simulink model "test_2"  (R2024b)
settings: Solver=FixedStepAuto  StartTime=0.0  StopTime=100000  RelTol=1e-3  EnableMultiTasking=on
undefined symbols (not defined in the file): BOOL, DINT, OTL, slplc
libraries: arduinolib x4
(part 1 of 8)
settings Model: ExtModeTrigDuration=2  Creator=Elliot  LastModifiedBy=Elliot
settings SolverCC: AutoInsertRateTranBlk=on
settings OptimizationCC: EnhancedBackFolding=on  PassReuseOutputArgsAs=Individual arguments  ZeroExternalMemoryAtStartup=off  ZeroInternalMemoryAtStartup=off  MaxStackSize=64  OptimizeBlockOrder=speed  DifferentSizesBufferReuse=on  OptimizationCustomize=off  EfficientTunableParamExpr=on
settings DebuggingCC: ParameterTunabilityLossMsg=error
settings HardwareCC: ProdBitPerInt=16  ProdBitPerPointer=16  ProdBitPerSizeT=16  ProdBitPerPtrDiffT=16  ProdLargestAtomicFloat=None  ProdWordSize=8  ProdHWDeviceType=Atmel->AVR
settings SFSimCC: MATLABDynamicMemAlloc=off
settings RTWCC: Description=Embedded Coder  SystemTargetFile=ert.tlc  HardwareBoard=Arduino Uno  TemplateMakefile=ert_default_tmf  Toolchain=Arduino AVR  BuildConfiguration=Faster Runs
settings CodeAppCC: ForceParamTrailComments=on  IgnoreCustomStorageClasses=off  OperatorAnnotations=on  SimulinkDataObjDesc=on  SFDataObjDesc=on  InsertBlockDesc=on
settings ERTTargetCC: SupportContinuousTime=on  SupportVariableSizeSignals=on  ExtModeTransport=3  ExtModeStaticAlloc=on  ExtModeAutomaticAllocSize=off  ExtModeStaticAllocSize=250  ExtModeMexFile=ext_xcp  ExtModeIntrfLevel=Level2 - Open  InlinedParameterPlacement=Hierarchical

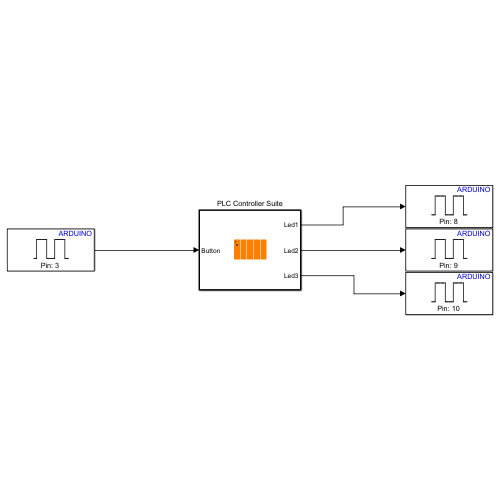
[thumbnail: Simulink's stored preview of the top-level diagram]
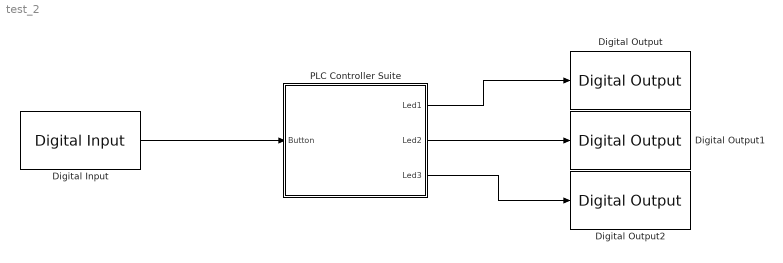
== system test_2 ==
  Digital Input : arduinolib/Digital Input  pinNumber=3  mode=Default  Direction=input  SampleTime=0.1  blockPlatform=arduino
  Digital Output : arduinolib/Digital Output  pinNumber=8  Direction=output  blockPlatform=arduino
  Digital Output1 : arduinolib/Digital Output  pinNumber=9  Direction=output  blockPlatform=arduino
  Digital Output2 : arduinolib/Digital Output  pinNumber=10  Direction=output  blockPlatform=arduino
  PLC Controller Suite : Subsystem  TreatAsAtomicUnit=on  mask{PLCBlockType=PLCController, PLCPOUType=PLC Controller}
      mask init:
      | slplc.callbacks.initController(gcb);
      settings: OpenFcn=slplc.callbacks.openPOUBlock(gcb);
      mask Help: web([docroot '/plccoder/ref/plccontrollersuite' '.html']);
      mask DialogControl PLCBlockTitle Prompt: PLC Controller Block
  wires:
  PLC Controller Suite/1(Led1) -> Digital Output/1
  PLC Controller Suite/2(Led2) -> Digital Output1/1
  PLC Controller Suite/3(Led3) -> Digital Output2/1
  Digital Input/1 -> PLC Controller Suite/1(Button)

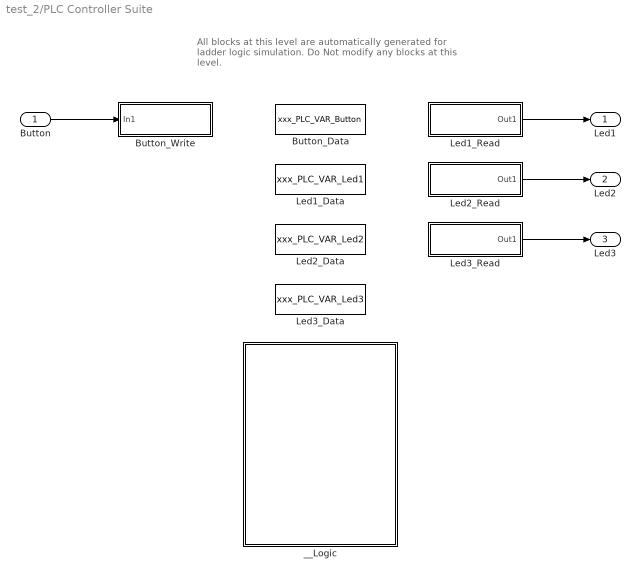
== system test_2/PLC Controller Suite ==
  note: All blocks at this level are automatically generated for ladder logic simulation.
      | Do Not modify any blocks at this level.
  Button : Inport  OutDataTypeStr=boolean
  Button_Data : DataStoreMemory  Tag=POUVariable  Priority=10  DataStoreName=xxx_PLC_VAR_Button  ShowAdditionalParam=off  OutDataTypeStr=boolean  Dimensions=1
  Button_Write : Subsystem  Priority=11  DisableCoverage=on  TreatAsAtomicUnit=on  mask{PLCOperandTag=Button, PLCOperandExpression=xxx_PLC_VAR_Button, PLCBlockType=VarWrite, PLCPOUType=VarWrite}
      mask prompts: PLCOperandTag "Operand Tag:"
      mask init:
      | slplc.callbacks.initInstruction(gcb);
      mask Help: web([docroot '/plccoder/ref/varwrite' '.html']);
      mask DialogControl PLCBlockTitle Prompt: Variable Write
      mask Display: disp(get_param(gcb, 'PLCOperandTag'));
  Led1_Data : DataStoreMemory  Tag=POUVariable  Priority=10  DataStoreName=xxx_PLC_VAR_Led1  ShowAdditionalParam=off  OutDataTypeStr=boolean  Dimensions=1
  Led1_Read : Subsystem  Priority=13  DisableCoverage=on  TreatAsAtomicUnit=on  mask{PLCOperandTag=Led1, PLCOperandExpression=xxx_PLC_VAR_Led1, PLCBlockType=VarRead, PLCPOUType=VarRead}
      mask prompts: PLCOperandTag "Operand Tag"
      mask init:
      | block = gcb;
      | maskObj = Simulink.Mask.get(block);
      | maskObj.Display = sprintf('disp(''%s'');', PLCOperandTag);
      | slplc.callbacks.initInstruction(gcb);
      mask Help: web([docroot '/plccoder/ref/varread' '.html']);
      mask DialogControl PLCBlockTitle Prompt: Variable Read
      mask Display: disp('Led1');
  Led2_Data : DataStoreMemory  Tag=POUVariable  Priority=10  DataStoreName=xxx_PLC_VAR_Led2  ShowAdditionalParam=off  OutDataTypeStr=boolean  Dimensions=1
  Led2_Read : Subsystem  Priority=13  DisableCoverage=on  TreatAsAtomicUnit=on  mask{PLCOperandTag=Led2, PLCOperandExpression=xxx_PLC_VAR_Led2, PLCBlockType=VarRead, PLCPOUType=VarRead}
      mask prompts: PLCOperandTag "Operand Tag"
      mask init:
      | block = gcb;
      | maskObj = Simulink.Mask.get(block);
      | maskObj.Display = sprintf('disp(''%s'');', PLCOperandTag);
      | slplc.callbacks.initInstruction(gcb);
      mask Help: web([docroot '/plccoder/ref/varread' '.html']);
      mask DialogControl PLCBlockTitle Prompt: Variable Read
      mask Display: disp('Led2');
  Led3_Data : DataStoreMemory  Tag=POUVariable  Priority=10  DataStoreName=xxx_PLC_VAR_Led3  ShowAdditionalParam=off  OutDataTypeStr=boolean  Dimensions=1
  Led3_Read : Subsystem  Priority=13  DisableCoverage=on  TreatAsAtomicUnit=on  mask{PLCOperandTag=Led3, PLCOperandExpression=xxx_PLC_VAR_Led3, PLCBlockType=VarRead, PLCPOUType=VarRead}
      mask prompts: PLCOperandTag "Operand Tag"
      mask init:
      | block = gcb;
      | maskObj = Simulink.Mask.get(block);
      | maskObj.Display = sprintf('disp(''%s'');', PLCOperandTag);
      | slplc.callbacks.initInstruction(gcb);
      mask Help: web([docroot '/plccoder/ref/varread' '.html']);
      mask DialogControl PLCBlockTitle Prompt: Variable Read
      mask Display: disp('Led3');
  __Logic : Subsystem  Priority=12  TreatAsAtomicUnit=on
  Led1 : Outport
  Led2 : Outport  Port=2
  Led3 : Outport  Port=3
  wires:
  Button/1 -> Button_Write/1(In1)
  Led1_Read/1(Out1) -> Led1/1
  Led2_Read/1(Out1) -> Led2/1
  Led3_Read/1(Out1) -> Led3/1

== system test_2/PLC Controller Suite/Button_Write ==
  In1 : Inport
  __CoreVarWrite : Subsystem  Tag=CoreVarWriteBlock  DisableCoverage=on  TreatAsAtomicUnit=on  mask{PLCBlockType=CoreVarWrite}
      mask init:
      | slplc.callbacks.initCoreVariable(gcb, 'write');
      mask DialogControl PLCBlockTitle Prompt: Core Variable Write
  wires:
  In1/1 -> __CoreVarWrite/1(u)

== system test_2/PLC Controller Suite/Led1_Read ==
  __CoreVarRead : Subsystem  Tag=CoreVarReadBlock  DisableCoverage=on  TreatAsAtomicUnit=on  mask{PLCBlockType=CoreVarRead}
      mask init:
      | slplc.callbacks.initCoreVariable(gcb, 'read');
      mask DialogControl PLCBlockTitle Prompt: Core Variable Read
  Out1 : Outport  VectorParamsAs1DForOutWhenUnconnected=off
  wires:
  __CoreVarRead/1(y) -> Out1/1

== system test_2/PLC Controller Suite/Led2_Read ==
  __CoreVarRead : Subsystem  Tag=CoreVarReadBlock  DisableCoverage=on  TreatAsAtomicUnit=on  mask{PLCBlockType=CoreVarRead}
      mask init:
      | slplc.callbacks.initCoreVariable(gcb, 'read');
      mask DialogControl PLCBlockTitle Prompt: Core Variable Read
  Out1 : Outport  VectorParamsAs1DForOutWhenUnconnected=off
  wires:
  __CoreVarRead/1(y) -> Out1/1

== system test_2/PLC Controller Suite/Led3_Read ==
  __CoreVarRead : Subsystem  Tag=CoreVarReadBlock  DisableCoverage=on  TreatAsAtomicUnit=on  mask{PLCBlockType=CoreVarRead}
      mask init:
      | slplc.callbacks.initCoreVariable(gcb, 'read');
      mask DialogControl PLCBlockTitle Prompt: Core Variable Read
  Out1 : Outport  VectorParamsAs1DForOutWhenUnconnected=off
  wires:
  __CoreVarRead/1(y) -> Out1/1

== system test_2/PLC Controller Suite/__Logic ==
  Controller Tags : Subsystem  Tag=ControllerVariableSS  DisableCoverage=on  TreatAsAtomicUnit=on  mask{PLCVarButtonName=Button, PLCVarButtonAddress=<empty>, PLCVarButtonMapping=Input Symbol, PLCVarButtonPortIndex=1, PLCVarButtonDataType=boolean, PLCVarButtonSize=1, PLCVarButtonInitialValue=0, PLCVarButtonToDelete=off, PLCVarLed1Name=Led1, PLCVarLed1Address=<empty>, PLCVarLed1Mapping=Output Symbol, PLCVarLed1PortIndex=1, PLCVarLed1DataType=boolean, PLCVarLed1Size=1, PLCVarLed1InitialValue=0, PLCVarLed1ToDelete=off, PLCVarLed2Name=Led2, PLCVarLed2Address=<empty>, PLCVarLed2Mapping=Output Symbol, PLCVarLed2PortIndex=2, PLCVarLed2DataType=boolean, PLCVarLed2Size=1, PLCVarLed2InitialValue=0, PLCVarLed2ToDelete=off, PLCVarLed3Name=Led3, PLCVarLed3Address=<empty>, PLCVarLed3Mapping=Output Symbol, PLCVarLed3PortIndex=3, PLCVarLed3DataType=boolean, PLCVarLed3Size=1, PLCVarLed3InitialValue=0, PLCVarLed3ToDelete=off}
      mask init:
      | slplc.callbacks.initControllerVarSS(gcb);
      settings: OpenFcn=slplc.callbacks.openControllerVariableSS(gcb);
      mask Help: web([docroot '/plccoder/ref/controllertags' '.html']);
      mask TypeOptions PLCVarButtonMapping: Global Variable | Input Symbol | Output Symbol
      mask TypeOptions PLCVarButtonPortIndex: 1 | 2 | 3 | 4
      mask TypeOptions PLCVarLed1Mapping: Global Variable | Input Symbol | Output Symbol
      mask TypeOptions PLCVarLed1PortIndex: 1 | 2 | 3 | 4
      mask TypeOptions PLCVarLed2Mapping: Global Variable | Input Symbol | Output Symbol
      mask TypeOptions PLCVarLed2PortIndex: 1 | 2 | 3 | 4
      mask TypeOptions PLCVarLed3Mapping: Global Variable | Input Symbol | Output Symbol
      mask TypeOptions PLCVarLed3PortIndex: 1 | 2 | 3 | 4
      mask DialogControl PLCBlockTitle Prompt: Global Variable and Symbol Spreadsheet
      mask DialogControl PLCVarListHeaderName Prompt: Name
      mask DialogControl PLCVarListHeaderAddress Prompt: Address (At)
      mask DialogControl PLCVarListHeaderMapping Prompt: Mapping Type
      mask DialogControl PLCVarListHeaderPortIndex Prompt: Port
      mask DialogControl PLCVarListHeaderDataType Prompt: Data Type
      mask DialogControl PLCVarListHeaderSize Prompt: Size
      mask DialogControl PLCVarListHeaderInitialValue Prompt: Initial Value
      mask DialogControl PLCVarListHeaderToDelete Prompt: Delete
  Task : Subsystem  TreatAsAtomicUnit=on  mask{PLCBlockType=Task, PLCPOUType=Task, PLCTaskWatchDog=0}
      settings: OpenFcn=slplc.callbacks.openTaskBlock(gcb);
      mask Help: web([docroot '/plccoder/ref/task' '.html']);
      mask DialogControl PLCBlockTitle Prompt: Task
  Up to Parent POU : Subsystem  DisableCoverage=on  TreatAsAtomicUnit=on  mask{PLCBlockType=OpenParentPOU}
      settings: OpenFcn=slplc.callbacks.openParentPOUBlock(gcb);
      mask Help: web([docroot '/plccoder/ref/uptoparentpou' '.html']);
      mask DialogControl PLCBlockTitle Prompt: Add Single Rung

== system test_2/PLC Controller Suite/Button_Write/__CoreVarWrite ==
  u : Inport
  DataWrite : DataStoreWrite  DataStoreName=xxx_PLC_VAR_Button  IndexOptions=Index vector (dialog)  Indices=1  OutputSizes=1
  wires:
  u/1 -> DataWrite/1

== system test_2/PLC Controller Suite/Led1_Read/__CoreVarRead ==
  DataRead : DataStoreRead  DataStoreName=xxx_PLC_VAR_Led1  IndexOptions=Index vector (dialog)  Indices=1  OutputSizes=1
  y : Outport  VectorParamsAs1DForOutWhenUnconnected=off
  wires:
  DataRead/1 -> y/1

== system test_2/PLC Controller Suite/Led2_Read/__CoreVarRead ==
  DataRead : DataStoreRead  DataStoreName=xxx_PLC_VAR_Led2  IndexOptions=Index vector (dialog)  Indices=1  OutputSizes=1
  y : Outport  VectorParamsAs1DForOutWhenUnconnected=off
  wires:
  DataRead/1 -> y/1

== system test_2/PLC Controller Suite/Led3_Read/__CoreVarRead ==
  DataRead : DataStoreRead  DataStoreName=xxx_PLC_VAR_Led3  IndexOptions=Index vector (dialog)  Indices=1  OutputSizes=1
  y : Outport  VectorParamsAs1DForOutWhenUnconnected=off
  wires:
  DataRead/1 -> y/1

== system test_2/PLC Controller Suite/__Logic/Controller Tags ==

== system test_2/PLC Controller Suite/__Logic/Task ==
  Program : Subsystem  TreatAsAtomicUnit=on  mask{PLCPOUType=Program, PLCPOULanguage=LD, PLCBlockType=LDProgram}
      mask prompts: PLCPOUType "POU Type:"
      mask init:
      | slplc.callbacks.initProgram(gcb);
      settings: OpenFcn=slplc.callbacks.openPOUBlock(gcb);
      mask Help: web([docroot '/plccoder/ref/ldprogram' '.html']);
      mask DialogControl PLCBlockTitle Prompt: Program
      mask DialogControl PLCEditPOU Prompt: Edit POU
      mask DialogControl PLCEditInterface Prompt: Edit Variables
  Up to Parent POU : Subsystem  DisableCoverage=on  TreatAsAtomicUnit=on  mask{PLCBlockType=OpenParentPOU}
      settings: OpenFcn=slplc.callbacks.openParentPOUBlock(gcb);
      mask Help: web([docroot '/plccoder/ref/uptoparentpou' '.html']);
      mask DialogControl PLCBlockTitle Prompt: Add Single Rung

== system test_2/PLC Controller Suite/__Logic/Up to Parent POU ==

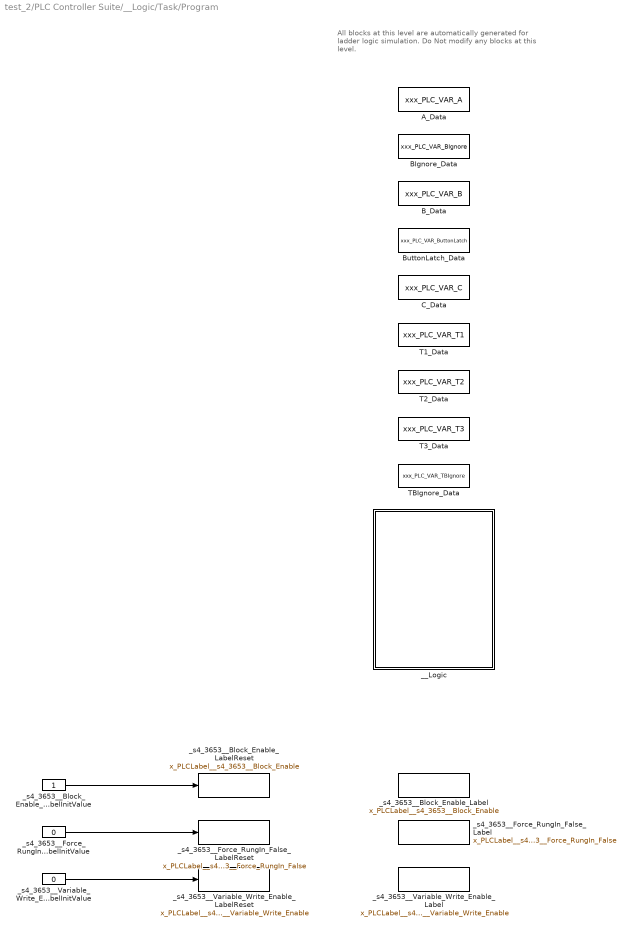
== system test_2/PLC Controller Suite/__Logic/Task/Program ==
  note: All blocks at this level are automatically generated for ladder logic simulation.
      | Do Not modify any blocks at this level.
  A_Data : DataStoreMemory  Tag=POUVariable  Priority=10  DataStoreName=xxx_PLC_VAR_A  InitialValue=true  ShowAdditionalParam=off  OutDataTypeStr=BOOL  Dimensions=1
  BIgnore_Data : DataStoreMemory  Tag=POUVariable  Priority=10  DataStoreName=xxx_PLC_VAR_BIgnore  InitialValue=false  ShowAdditionalParam=off  OutDataTypeStr=BOOL  Dimensions=1
  B_Data : DataStoreMemory  Tag=POUVariable  Priority=10  DataStoreName=xxx_PLC_VAR_B  InitialValue=false  ShowAdditionalParam=off  OutDataTypeStr=BOOL  Dimensions=1
  ButtonLatch_Data : DataStoreMemory  Tag=POUVariable  Priority=10  DataStoreName=xxx_PLC_VAR_ButtonLatch  InitialValue=false  ShowAdditionalParam=off  OutDataTypeStr=BOOL  Dimensions=1
  C_Data : DataStoreMemory  Tag=POUVariable  Priority=10  DataStoreName=xxx_PLC_VAR_C  InitialValue=false  ShowAdditionalParam=off  OutDataTypeStr=BOOL  Dimensions=1
  T1_Data : DataStoreMemory  Tag=POUVariable  Priority=10  DataStoreName=xxx_PLC_VAR_T1  InitialValue=T1_InitialValue  ShowAdditionalParam=off  OutDataTypeStr=Bus: TIMER  Dimensions=1
  T2_Data : DataStoreMemory  Tag=POUVariable  Priority=10  DataStoreName=xxx_PLC_VAR_T2  InitialValue=T1_InitialValue  ShowAdditionalParam=off  OutDataTypeStr=Bus: TIMER  Dimensions=1
  T3_Data : DataStoreMemory  Tag=POUVariable  Priority=10  DataStoreName=xxx_PLC_VAR_T3  InitialValue=T1_InitialValue  ShowAdditionalParam=off  OutDataTypeStr=Bus: TIMER  Dimensions=1
  TBIgnore_Data : DataStoreMemory  Tag=POUVariable  Priority=10  DataStoreName=xxx_PLC_VAR_TBIgnore  InitialValue=T2_InitialValue  ShowAdditionalParam=off  OutDataTypeStr=Bus: TIMER  Dimensions=1
  __Logic : Subsystem  Priority=12  TreatAsAtomicUnit=on
  _s4_3653__Block_Enable_Label : DataStoreMemory  Priority=10  DataStoreName=x_PLCLabel__s4_3653__Block_Enable  InitialValue=1  ShowAdditionalParam=off  OutDataTypeStr=BOOL  Dimensions=1
  _s4_3653__Block_Enable_LabelInitValue : Constant  OutDataTypeStr=BOOL
  _s4_3653__Block_Enable_LabelReset : DataStoreWrite  Priority=11  DataStoreName=x_PLCLabel__s4_3653__Block_Enable  IndexOptions=Index vector (dialog)  Indices=1  OutputSizes=1
  _s4_3653__Force_RungIn_False_Label : DataStoreMemory  Priority=10  DataStoreName=x_PLCLabel__s4_3653__Force_RungIn_False  ShowAdditionalParam=off  OutDataTypeStr=BOOL  Dimensions=1
  _s4_3653__Force_RungIn_False_LabelInitValue : Constant  Value=0  OutDataTypeStr=BOOL
  _s4_3653__Force_RungIn_False_LabelReset : DataStoreWrite  Priority=11  DataStoreName=x_PLCLabel__s4_3653__Force_RungIn_False  IndexOptions=Index vector (dialog)  Indices=1  OutputSizes=1
  _s4_3653__Variable_Write_Enable_Label : DataStoreMemory  Priority=10  DataStoreName=x_PLCLabel__s4_3653__Variable_Write_Enable  ShowAdditionalParam=off  OutDataTypeStr=BOOL  Dimensions=1
  _s4_3653__Variable_Write_Enable_LabelInitValue : Constant  Value=0  OutDataTypeStr=BOOL
  _s4_3653__Variable_Write_Enable_LabelReset : DataStoreWrite  Priority=11  DataStoreName=x_PLCLabel__s4_3653__Variable_Write_Enable  IndexOptions=Index vector (dialog)  Indices=1  OutputSizes=1
  wires:
  _s4_3653__Block_Enable_LabelInitValue/1 -> _s4_3653__Block_Enable_LabelReset/1
  _s4_3653__Variable_Write_Enable_LabelInitValue/1 -> _s4_3653__Variable_Write_Enable_LabelReset/1
  _s4_3653__Force_RungIn_False_LabelInitValue/1 -> _s4_3653__Force_RungIn_False_LabelReset/1

== system test_2/PLC Controller Suite/__Logic/Task/Up to Parent POU ==

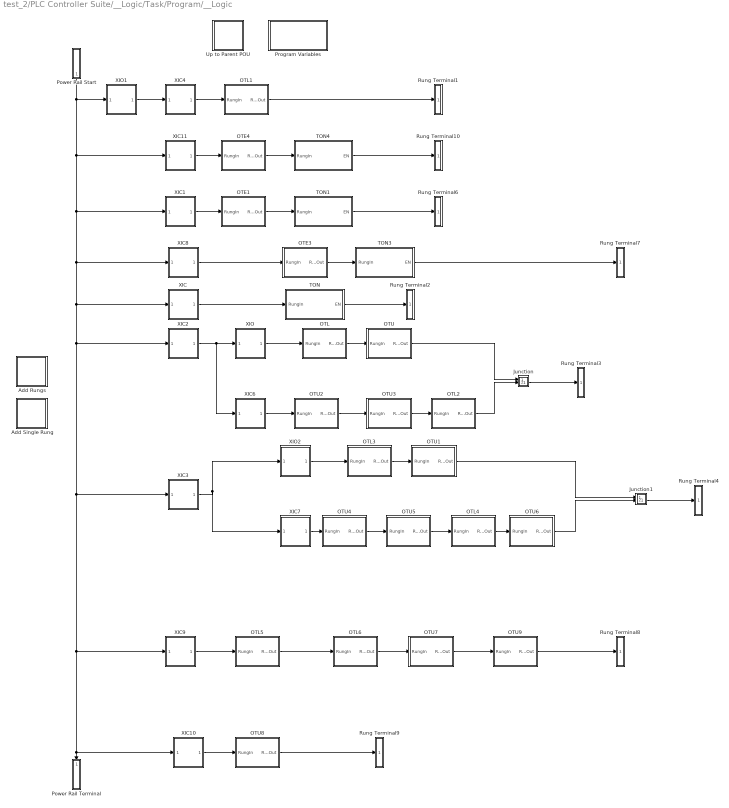
== system test_2/PLC Controller Suite/__Logic/Task/Program/__Logic ==
  Add Rungs : Subsystem  DisableCoverage=on  TreatAsAtomicUnit=on  mask{PLCRungNumberToAdd=1, PLCBlockType=AddRungs}
      mask prompts: PLCRungNumberToAdd "Rung Number:"
      mask Help: web([docroot '/plccoder/ref/addrungs' '.html']);
      mask DialogControl PLCAddRungs Prompt: Add Rungs
      mask DialogControl PLCRungAddButton Prompt: Add
      mask DialogControl PLCRungAddButton Callback: slplc.callbacks.addLadderRungs(gcb);
      mask Display: disp(sprintf(['Add' newline 'Rungs']));
  Add Single Rung : Subsystem  DisableCoverage=on  TreatAsAtomicUnit=on  mask{PLCRungNumberToAdd=1, PLCBlockType=AddSingleRung}
      settings: OpenFcn=slplc.callbacks.addLadderRungs(gcb);
      mask Help: web([docroot '/plccoder/ref/addsinglerung' '.html']);
      mask DialogControl PLCAddRung Prompt: Add Single Rung
      mask Display: disp(sprintf(['Add' newline '1 Rung']));
  Junction : Subsystem  Priority=29  DisableCoverage=on  TreatAsAtomicUnit=on  mask{PLCBlockType=Junction, PLCPOUType=BranchJunction}
      mask Help: web([docroot '/plccoder/ref/junction' '.html']);
      mask DialogControl PLCBlockTitle Prompt: Rung Merge Point
      mask DialogControl PLCBlockDesc Prompt: This is the ladder diagram rung merge point.
  Junction1 : Subsystem  Priority=40  DisableCoverage=on  TreatAsAtomicUnit=on  mask{PLCBlockType=Junction, PLCPOUType=BranchJunction}
      mask Help: web([docroot '/plccoder/ref/junction' '.html']);
      mask DialogControl PLCBlockTitle Prompt: Rung Merge Point
      mask DialogControl PLCBlockDesc Prompt: This is the ladder diagram rung merge point.
  OTE1 : Subsystem  Priority=11  TreatAsAtomicUnit=on  mask{PLCOperandTag=Led2, PLCBlockType=OTE, PLCPOUType=Coil, PLCOperandExpression=xxx_PLC_VAR_Led2}
      mask prompts: PLCOperandTag "Operand Tag:"
      mask init:
      | slplc.callbacks.initInstruction(gcb);
      settings: AttributesFormatString=%<PLCOperandTag>
      mask Help: web([docroot '/plccoder/ref/ote' '.html']);
      mask DialogControl PLCBlockTitle Prompt: Output Energize (OTE)
  OTE3 : Subsystem  Priority=15  TreatAsAtomicUnit=on  mask{PLCOperandTag=Led3, PLCBlockType=OTE, PLCPOUType=Coil, PLCOperandExpression=xxx_PLC_VAR_Led3}
      mask prompts: PLCOperandTag "Operand Tag:"
      mask init:
      | slplc.callbacks.initInstruction(gcb);
      settings: AttributesFormatString=%<PLCOperandTag>
      mask Help: web([docroot '/plccoder/ref/ote' '.html']);
      mask DialogControl PLCBlockTitle Prompt: Output Energize (OTE)
  OTE4 : Subsystem  Priority=7  TreatAsAtomicUnit=on  mask{PLCOperandTag=Led1, PLCBlockType=OTE, PLCPOUType=Coil, PLCOperandExpression=xxx_PLC_VAR_Led1}
      mask prompts: PLCOperandTag "Operand Tag:"
      mask init:
      | slplc.callbacks.initInstruction(gcb);
      settings: AttributesFormatString=%<PLCOperandTag>
      mask Help: web([docroot '/plccoder/ref/ote' '.html']);
      mask DialogControl PLCBlockTitle Prompt: Output Energize (OTE)
  OTL : Subsystem  Priority=23  TreatAsAtomicUnit=on  mask{PLCOperandTag=B, PLCBlockType=OTL, PLCPOUType=Coil, PLCOperandExpression=xxx_PLC_VAR_B}
      mask prompts: PLCOperandTag "Operand Tag:"
      mask init:
      | slplc.callbacks.initInstruction(gcb);
      settings: AttributesFormatString=%<PLCOperandTag>
      mask Help: web([docroot '/plccoder/ref/otl' '.html']);
      mask DialogControl PLCBlockTitle Prompt: Output Latch (OTL)
      mask Display: disp('L');
  OTL1 : Subsystem  Priority=4  TreatAsAtomicUnit=on  mask{PLCOperandTag=ButtonLatch, PLCBlockType=OTL, PLCPOUType=Coil, PLCOperandExpression=xxx_PLC_VAR_ButtonLatch}
      mask prompts: PLCOperandTag "Operand Tag:"
      mask init:
      | slplc.callbacks.initInstruction(gcb);
      settings: AttributesFormatString=%<PLCOperandTag>
      mask Help: web([docroot '/plccoder/ref/otl' '.html']);
      mask DialogControl PLCBlockTitle Prompt: Output Latch (OTL)
      mask Display: disp('L');
  OTL2 : Subsystem  Priority=28  TreatAsAtomicUnit=on  mask{PLCOperandTag=C, PLCBlockType=OTL, PLCPOUType=Coil, PLCOperandExpression=xxx_PLC_VAR_C}
      mask prompts: PLCOperandTag "Operand Tag:"
      mask init:
      | slplc.callbacks.initInstruction(gcb);
      settings: AttributesFormatString=%<PLCOperandTag>
      mask Help: web([docroot '/plccoder/ref/otl' '.html']);
      mask DialogControl PLCBlockTitle Prompt: Output Latch (OTL)
      mask Display: disp('L');
  OTL3 : Subsystem  Priority=33  TreatAsAtomicUnit=on  mask{PLCOperandTag=A, PLCBlockType=OTL, PLCPOUType=Coil, PLCOperandExpression=xxx_PLC_VAR_A}
      mask prompts: PLCOperandTag "Operand Tag:"
      mask init:
      | slplc.callbacks.initInstruction(gcb);
      settings: AttributesFormatString=%<PLCOperandTag>
      mask Help: web([docroot '/plccoder/ref/otl' '.html']);
      mask DialogControl PLCBlockTitle Prompt: Output Latch (OTL)
      mask Display: disp('L');
  OTL4 : Subsystem  Priority=38  TreatAsAtomicUnit=on  mask{PLCOperandTag=C, PLCBlockType=OTL, PLCPOUType=Coil, PLCOperandExpression=xxx_PLC_VAR_C}
      mask prompts: PLCOperandTag "Operand Tag:"
      mask init:
      | slplc.callbacks.initInstruction(gcb);
      settings: AttributesFormatString=%<PLCOperandTag>
      mask Help: web([docroot '/plccoder/ref/otl' '.html']);
      mask DialogControl PLCBlockTitle Prompt: Output Latch (OTL)
      mask Display: disp('L');
  OTL5 : Subsystem  Priority=43  TreatAsAtomicUnit=on  mask{PLCOperandTag=A, PLCBlockType=OTL, PLCPOUType=Coil, PLCOperandExpression=xxx_PLC_VAR_A}
      mask prompts: PLCOperandTag "Operand Tag:"
      mask init:
      | slplc.callbacks.initInstruction(gcb);
      settings: AttributesFormatString=%<PLCOperandTag>
      mask Help: web([docroot '/plccoder/ref/otl' '.html']);
      mask DialogControl PLCBlockTitle Prompt: Output Latch (OTL)
      mask Display: disp('L');
  OTL6 : Subsystem  Priority=44  TreatAsAtomicUnit=on  mask{PLCOperandTag=BIgnore, PLCBlockType=OTL, PLCPOUType=Coil, PLCOperandExpression=xxx_PLC_VAR_BIgnore}
      mask prompts: PLCOperandTag "Operand Tag:"
      mask init:
      | slplc.callbacks.initInstruction(gcb);
      settings: AttributesFormatString=%<PLCOperandTag>
      mask Help: web([docroot '/plccoder/ref/otl' '.html']);
      mask DialogControl PLCBlockTitle Prompt: Output Latch (OTL)
      mask Display: disp('L');
  OTU : Subsystem  Priority=24  TreatAsAtomicUnit=on  mask{PLCOperandTag=A, PLCBlockType=OTU, PLCPOUType=Coil, PLCOperandExpression=xxx_PLC_VAR_A}
      mask prompts: PLCOperandTag "Operand Tag:"
      mask init:
      | slplc.callbacks.initInstruction(gcb);
      settings: AttributesFormatString=%<PLCOperandTag>
      mask Help: web([docroot '/plccoder/ref/otu' '.html']);
      mask DialogControl PLCBlockTitle Prompt: Output Unlatch (OTU)
      mask Display: disp('U');
  OTU1 : Subsystem  Priority=34  TreatAsAtomicUnit=on  mask{PLCOperandTag=B, PLCBlockType=OTU, PLCPOUType=Coil, PLCOperandExpression=xxx_PLC_VAR_B}
      mask prompts: PLCOperandTag "Operand Tag:"
      mask init:
      | slplc.callbacks.initInstruction(gcb);
      settings: AttributesFormatString=%<PLCOperandTag>
      mask Help: web([docroot '/plccoder/ref/otu' '.html']);
      mask DialogControl PLCBlockTitle Prompt: Output Unlatch (OTU)
      mask Display: disp('U');
  OTU2 : Subsystem  Priority=26  TreatAsAtomicUnit=on  mask{PLCOperandTag=A, PLCBlockType=OTU, PLCPOUType=Coil, PLCOperandExpression=xxx_PLC_VAR_A}
      mask prompts: PLCOperandTag "Operand Tag:"
      mask init:
      | slplc.callbacks.initInstruction(gcb);
      settings: AttributesFormatString=%<PLCOperandTag>
      mask Help: web([docroot '/plccoder/ref/otu' '.html']);
      mask DialogControl PLCBlockTitle Prompt: Output Unlatch (OTU)
      mask Display: disp('U');
  OTU3 : Subsystem  Priority=27  TreatAsAtomicUnit=on  mask{PLCOperandTag=B, PLCBlockType=OTU, PLCPOUType=Coil, PLCOperandExpression=xxx_PLC_VAR_B}
      mask prompts: PLCOperandTag "Operand Tag:"
      mask init:
      | slplc.callbacks.initInstruction(gcb);
      settings: AttributesFormatString=%<PLCOperandTag>
      mask Help: web([docroot '/plccoder/ref/otu' '.html']);
      mask DialogControl PLCBlockTitle Prompt: Output Unlatch (OTU)
      mask Display: disp('U');
  OTU4 : Subsystem  Priority=36  TreatAsAtomicUnit=on  mask{PLCOperandTag=A, PLCBlockType=OTU, PLCPOUType=Coil, PLCOperandExpression=xxx_PLC_VAR_A}
      mask prompts: PLCOperandTag "Operand Tag:"
      mask init:
      | slplc.callbacks.initInstruction(gcb);
      settings: AttributesFormatString=%<PLCOperandTag>
      mask Help: web([docroot '/plccoder/ref/otu' '.html']);
      mask DialogControl PLCBlockTitle Prompt: Output Unlatch (OTU)
      mask Display: disp('U');
  OTU5 : Subsystem  Priority=37  TreatAsAtomicUnit=on  mask{PLCOperandTag=B, PLCBlockType=OTU, PLCPOUType=Coil, PLCOperandExpression=xxx_PLC_VAR_B}
      mask prompts: PLCOperandTag "Operand Tag:"
      mask init:
      | slplc.callbacks.initInstruction(gcb);
      settings: AttributesFormatString=%<PLCOperandTag>
      mask Help: web([docroot '/plccoder/ref/otu' '.html']);
      mask DialogControl PLCBlockTitle Prompt: Output Unlatch (OTU)
      mask Display: disp('U');
  OTU6 : Subsystem  Priority=39  TreatAsAtomicUnit=on  mask{PLCOperandTag=ButtonLatch, PLCBlockType=OTU, PLCPOUType=Coil, PLCOperandExpression=xxx_PLC_VAR_ButtonLatch}
      mask prompts: PLCOperandTag "Operand Tag:"
      mask init:
      | slplc.callbacks.initInstruction(gcb);
      settings: AttributesFormatString=%<PLCOperandTag>
      mask Help: web([docroot '/plccoder/ref/otu' '.html']);
      mask DialogControl PLCBlockTitle Prompt: Output Unlatch (OTU)
      mask Display: disp('U');
  OTU7 : Subsystem  Priority=45  TreatAsAtomicUnit=on  mask{PLCOperandTag=ButtonLatch, PLCBlockType=OTU, PLCPOUType=Coil, PLCOperandExpression=xxx_PLC_VAR_ButtonLatch}
      mask prompts: PLCOperandTag "Operand Tag:"
      mask init:
      | slplc.callbacks.initInstruction(gcb);
      settings: AttributesFormatString=%<PLCOperandTag>
      mask Help: web([docroot '/plccoder/ref/otu' '.html']);
      mask DialogControl PLCBlockTitle Prompt: Output Unlatch (OTU)
      mask Display: disp('U');
  OTU8 : Subsystem  Priority=49  TreatAsAtomicUnit=on  mask{PLCOperandTag=BIgnore, PLCBlockType=OTU, PLCPOUType=Coil, PLCOperandExpression=xxx_PLC_VAR_BIgnore}
      mask prompts: PLCOperandTag "Operand Tag:"
      mask init:
      | slplc.callbacks.initInstruction(gcb);
      settings: AttributesFormatString=%<PLCOperandTag>
      mask Help: web([docroot '/plccoder/ref/otu' '.html']);
      mask DialogControl PLCBlockTitle Prompt: Output Unlatch (OTU)
      mask Display: disp('U');
  OTU9 : Subsystem  Priority=46  TreatAsAtomicUnit=on  mask{PLCOperandTag=C, PLCBlockType=OTU, PLCPOUType=Coil, PLCOperandExpression=xxx_PLC_VAR_C}
      mask prompts: PLCOperandTag "Operand Tag:"
      mask init:
      | slplc.callbacks.initInstruction(gcb);
      settings: AttributesFormatString=%<PLCOperandTag>
      mask Help: web([docroot '/plccoder/ref/otu' '.html']);
      mask DialogControl PLCBlockTitle Prompt: Output Unlatch (OTU)
      mask Display: disp('U');
  Power Rail Start : Subsystem  Priority=1  DisableCoverage=on  TreatAsAtomicUnit=on  mask{PLCBlockType=PowerRailStart}
      mask Help: web([docroot '/plccoder/ref/powerrailstart' '.html']);
      mask DialogControl PLCBlockTitle Prompt: Power Rail Start
      mask DialogControl PLCBlockDesc Prompt: This is the ladder diagram left power rail start block.
  Power Rail Terminal : Subsystem  DisableCoverage=on  TreatAsAtomicUnit=on  mask{PLCBlockType=PowerRailTerminal}
      mask Help: web([docroot '/plccoder/ref/powerrailterminal' '.html']);
      mask DialogControl PLCBlockTitle Prompt: Power Rail Terminal
      mask DialogControl PLCBlockDesc Prompt: This is the ladder diagram left power rail terminal block.
  Program Variables : Subsystem  Tag=ProgramVariableSS  DisableCoverage=on  TreatAsAtomicUnit=on  mask{PLCVarAName=A, PLCVarAScope=Local, PLCVarAPortType=Hidden, PLCVarAPortIndex=13, PLCVarADataType=BOOL, PLCVarASize=1, PLCVarAInitialValue=true, PLCVarAToDelete=off, PLCVarBName=B, PLCVarBScope=Local, PLCVarBPortType=Hidden, PLCVarBPortIndex=13, PLCVarBDataType=BOOL, PLCVarBSize=1, PLCVarBInitialValue=false, PLCVarBToDelete=off, PLCVarBIgnoreName=BIgnore, PLCVarBIgnoreScope=Local, PLCVarBIgnorePortType=Hidden, PLCVarBIgnorePortIndex=13, PLCVarBIgnoreDataType=BOOL, PLCVarBIgnoreSize=1, PLCVarBIgnoreInitialValue=false, PLCVarBIgnoreToDelete=off, PLCVarButtonLatchName=ButtonLatch, PLCVarButtonLatchScope=Local, PLCVarButtonLatchPortType=Hidden, PLCVarButtonLatchPortIndex=13, PLCVarButtonLatchDataType=BOOL, PLCVarButtonLatchSize=1, PLCVarButtonLatchInitialValue=false, PLCVarButtonLatchToDelete=off, PLCVarCName=C, PLCVarCScope=Local, PLCVarCPortType=Hidden, PLCVarCPortIndex=13, PLCVarCDataType=BOOL, PLCVarCSize=1, PLCVarCInitialValue=false, PLCVarCToDelete=off, PLCVarT1Name=T1, PLCVarT1Scope=Local, PLCVarT1PortType=Hidden, PLCVarT1PortIndex=13, PLCVarT1DataType=Bus: TIMER, PLCVarT1Size=1, PLCVarT1InitialValue=T1_InitialValue, PLCVarT1ToDelete=off, PLCVarT2Name=T2, PLCVarT2Scope=Local, PLCVarT2PortType=Hidden, PLCVarT2PortIndex=13, PLCVarT2DataType=Bus: TIMER, PLCVarT2Size=1, PLCVarT2InitialValue=T1_InitialValue, PLCVarT2ToDelete=off, PLCVarT3Name=T3, PLCVarT3Scope=Local, PLCVarT3PortType=Hidden, PLCVarT3PortIndex=13, PLCVarT3DataType=Bus: TIMER, PLCVarT3Size=1, PLCVarT3InitialValue=T1_InitialValue, PLCVarT3ToDelete=off, PLCVarTBIgnoreName=TBIgnore, PLCVarTBIgnoreScope=Local, PLCVarTBIgnorePortType=Hidden, PLCVarTBIgnorePortIndex=13, PLCVarTBIgnoreDataType=Bus: TIMER, PLCVarTBIgnoreSize=1, PLCVarTBIgnoreInitialValue=T2_InitialValue, PLCVarTBIgnoreToDelete=off, PLCVarButtonName=Button, PLCVarButtonScope=External, PLCVarButtonPortType=Hidden, PLCVarButtonPortIndex=13, PLCVarButtonDataType=DINT, PLCVarButtonSize=-1, PLCVarButtonInitialValue=0, PLCVarButtonToDelete=off, PLCVarLed1Name=Led1, PLCVarLed1Scope=External, PLCVarLed1PortType=Hidden, PLCVarLed1PortIndex=13, PLCVarLed1DataType=DINT, PLCVarLed1Size=-1, PLCVarLed1InitialValue=0, PLCVarLed1ToDelete=off, PLCVarLed2Name=Led2, PLCVarLed2Scope=External, PLCVarLed2PortType=Hidden, PLCVarLed2PortIndex=13, PLCVarLed2DataType=DINT, PLCVarLed2Size=-1, PLCVarLed2InitialValue=0, PLCVarLed2ToDelete=off, PLCVarLed3Name=Led3, PLCVarLed3Scope=External, PLCVarLed3PortType=Hidden, PLCVarLed3PortIndex=13, PLCVarLed3DataType=DINT, PLCVarLed3Size=-1, PLCVarLed3InitialValue=0, PLCVarLed3ToDelete=off}
      mask init:
      | slplc.callbacks.initPOUVarSS(gcb);
      settings: OpenFcn=slplc.callbacks.openProgramVariableSS(gcb);
      mask Help: web([docroot '/plccoder/ref/programvariables' '.html']);
      mask TypeOptions PLCVarAScope: Local | External
      mask TypeOptions PLCVarAPortType: Hidden | Inport | Outport
      mask TypeOptions PLCVarAPortIndex: 1 | 2 | 3 | 4 | 5 | 6 | 7 | 8 | 9 | 10 | 11 | 12 | 13
      mask TypeOptions PLCVarBScope: Local | External
      mask TypeOptions PLCVarBPortType: Hidden | Inport | Outport
      mask TypeOptions PLCVarBPortIndex: 1 | 2 | 3 | 4 | 5 | 6 | 7 | 8 | 9 | 10 | 11 | 12 | 13
      mask TypeOptions PLCVarBIgnoreScope: Local | External
      mask TypeOptions PLCVarBIgnorePortType: Hidden | Inport | Outport
      mask TypeOptions PLCVarBIgnorePortIndex: 1 | 2 | 3 | 4 | 5 | 6 | 7 | 8 | 9 | 10 | 11 | 12 | 13
      mask TypeOptions PLCVarButtonLatchScope: Local | External
      mask TypeOptions PLCVarButtonLatchPortType: Hidden | Inport | Outport
      mask TypeOptions PLCVarButtonLatchPortIndex: 1 | 2 | 3 | 4 | 5 | 6 | 7 | 8 | 9 | 10 | 11 | 12 | 13
      mask TypeOptions PLCVarCScope: Local | External
      mask TypeOptions PLCVarCPortType: Hidden | Inport | Outport
      mask TypeOptions PLCVarCPortIndex: 1 | 2 | 3 | 4 | 5 | 6 | 7 | 8 | 9 | 10 | 11 | 12 | 13
      mask TypeOptions PLCVarT1Scope: Local | External
      mask TypeOptions PLCVarT1PortType: Hidden | Inport | Outport
      mask TypeOptions PLCVarT1PortIndex: 1 | 2 | 3 | 4 | 5 | 6 | 7 | 8 | 9 | 10 | 11 | 12 | 13
      mask TypeOptions PLCVarT2Scope: Local | External
      mask TypeOptions PLCVarT2PortType: Hidden | Inport | Outport
      mask TypeOptions PLCVarT2PortIndex: 1 | 2 | 3 | 4 | 5 | 6 | 7 | 8 | 9 | 10 | 11 | 12 | 13
      mask TypeOptions PLCVarT3Scope: Local | External
      mask TypeOptions PLCVarT3PortType: Hidden | Inport | Outport
      mask TypeOptions PLCVarT3PortIndex: 1 | 2 | 3 | 4 | 5 | 6 | 7 | 8 | 9 | 10 | 11 | 12 | 13
      mask TypeOptions PLCVarTBIgnoreScope: Local | External
      mask TypeOptions PLCVarTBIgnorePortType: Hidden | Inport | Outport
      mask TypeOptions PLCVarTBIgnorePortIndex: 1 | 2 | 3 | 4 | 5 | 6 | 7 | 8 | 9 | 10 | 11 | 12 | 13
      mask TypeOptions PLCVarButtonScope: Local | External
      mask TypeOptions PLCVarButtonPortType: Hidden | Inport | Outport
      mask TypeOptions PLCVarButtonPortIndex: 1 | 2 | 3 | 4 | 5 | 6 | 7 | 8 | 9 | 10 | 11 | 12 | 13
      mask TypeOptions PLCVarLed1Scope: Local | External
      mask TypeOptions PLCVarLed1PortType: Hidden | Inport | Outport
      mask TypeOptions PLCVarLed1PortIndex: 1 | 2 | 3 | 4 | 5 | 6 | 7 | 8 | 9 | 10 | 11 | 12 | 13
      mask TypeOptions PLCVarLed2Scope: Local | External
      mask TypeOptions PLCVarLed2PortType: Hidden | Inport | Outport
      mask TypeOptions PLCVarLed2PortIndex: 1 | 2 | 3 | 4 | 5 | 6 | 7 | 8 | 9 | 10 | 11 | 12 | 13
      mask TypeOptions PLCVarLed3Scope: Local | External
      mask TypeOptions PLCVarLed3PortType: Hidden | Inport | Outport
      mask TypeOptions PLCVarLed3PortIndex: 1 | 2 | 3 | 4 | 5 | 6 | 7 | 8 | 9 | 10 | 11 | 12 | 13
      mask DialogControl PLCBlockTitle Prompt: Program Variable Spreadsheet
      mask DialogControl PLCVarListHeaderName Prompt: Name
      mask DialogControl PLCVarListHeaderScope Prompt: Scope
      mask DialogControl PLCVarListHeaderDataType Prompt: Data Type
      mask DialogControl PLCVarListHeaderSize Prompt: Size
      mask DialogControl PLCVarListHeaderInitialValue Prompt: Initial Value
      mask DialogControl PLCVarListHeaderToDelete Prompt: Delete
  Rung Terminal1 : Subsystem  Priority=5  DisableCoverage=on  TreatAsAtomicUnit=on  mask{PLCRungTerminalIndex=1, PLCBlockType=RungTerminal}
      settings: AttributesFormatString=Rung %<PLCRungTerminalIndex>
      mask Help: web([docroot '/plccoder/ref/rungterminal' '.html']);
      mask DialogControl PLCBlockTitle Prompt: Rung Terminal
      mask DialogControl PLCBlockDescText Prompt: This is the ladder diagram rung terminal.
  Rung Terminal10 : Subsystem  Priority=9  DisableCoverage=on  TreatAsAtomicUnit=on  mask{PLCRungTerminalIndex=2, PLCBlockType=RungTerminal}
      settings: AttributesFormatString=Rung %<PLCRungTerminalIndex>
      mask Help: web([docroot '/plccoder/ref/rungterminal' '.html']);
      mask DialogControl PLCBlockTitle Prompt: Rung Terminal
      mask DialogControl PLCBlockDescText Prompt: This is the ladder diagram rung terminal.
  Rung Terminal2 : Subsystem  Priority=20  DisableCoverage=on  TreatAsAtomicUnit=on  mask{PLCRungTerminalIndex=5, PLCBlockType=RungTerminal}
      settings: AttributesFormatString=Rung %<PLCRungTerminalIndex>
      mask Help: web([docroot '/plccoder/ref/rungterminal' '.html']);
      mask DialogControl PLCBlockTitle Prompt: Rung Terminal
      mask DialogControl PLCBlockDescText Prompt: This is the ladder diagram rung terminal.
  Rung Terminal3 : Subsystem  Priority=30  DisableCoverage=on  TreatAsAtomicUnit=on  mask{PLCRungTerminalIndex=6, PLCBlockType=RungTerminal}
      settings: AttributesFormatString=Rung %<PLCRungTerminalIndex>
      mask Help: web([docroot '/plccoder/ref/rungterminal' '.html']);
      mask DialogControl PLCBlockTitle Prompt: Rung Terminal
      mask DialogControl PLCBlockDescText Prompt: This is the ladder diagram rung terminal.
  Rung Terminal4 : Subsystem  Priority=41  DisableCoverage=on  TreatAsAtomicUnit=on  mask{PLCRungTerminalIndex=7, PLCBlockType=RungTerminal}
      settings: AttributesFormatString=Rung %<PLCRungTerminalIndex>
      mask Help: web([docroot '/plccoder/ref/rungterminal' '.html']);
      mask DialogControl PLCBlockTitle Prompt: Rung Terminal
      mask DialogControl PLCBlockDescText Prompt: This is the ladder diagram rung terminal.
  Rung Terminal6 : Subsystem  Priority=13  DisableCoverage=on  TreatAsAtomicUnit=on  mask{PLCRungTerminalIndex=3, PLCBlockType=RungTerminal}
      settings: AttributesFormatString=Rung %<PLCRungTerminalIndex>
      mask Help: web([docroot '/plccoder/ref/rungterminal' '.html']);
      mask DialogControl PLCBlockTitle Prompt: Rung Terminal
      mask DialogControl PLCBlockDescText Prompt: This is the ladder diagram rung terminal.
  Rung Terminal7 : Subsystem  Priority=17  DisableCoverage=on  TreatAsAtomicUnit=on  mask{PLCRungTerminalIndex=4, PLCBlockType=RungTerminal}
      settings: AttributesFormatString=Rung %<PLCRungTerminalIndex>
      mask Help: web([docroot '/plccoder/ref/rungterminal' '.html']);
      mask DialogControl PLCBlockTitle Prompt: Rung Terminal
      mask DialogControl PLCBlockDescText Prompt: This is the ladder diagram rung terminal.
  Rung Terminal8 : Subsystem  Priority=47  DisableCoverage=on  TreatAsAtomicUnit=on  mask{PLCRungTerminalIndex=8, PLCBlockType=RungTerminal}
      settings: AttributesFormatString=Rung %<PLCRungTerminalIndex>
      mask Help: web([docroot '/plccoder/ref/rungterminal' '.html']);
      mask DialogControl PLCBlockTitle Prompt: Rung Terminal
      mask DialogControl PLCBlockDescText Prompt: This is the ladder diagram rung terminal.
  Rung Terminal9 : Subsystem  Priority=50  DisableCoverage=on  TreatAsAtomicUnit=on  mask{PLCRungTerminalIndex=9, PLCBlockType=RungTerminal}
      settings: AttributesFormatString=Rung %<PLCRungTerminalIndex>
      mask Help: web([docroot '/plccoder/ref/rungterminal' '.html']);
      mask DialogControl PLCBlockTitle Prompt: Rung Terminal
      mask DialogControl PLCBlockDescText Prompt: This is the ladder diagram rung terminal.
  TON : Subsystem  Priority=19  TreatAsAtomicUnit=on  mask{PLCOperandTag=TBIgnore, PLCTimerSampleTime=2000, PLCBlockType=TON, PLCPOUType=stdFB, PLCOperandAccess=ReadWrite, PLCOperandExpression=xxx_PLC_VAR_TBIgnore}
      mask prompts: PLCOperandTag "Timer Tag:"; PLCTimerSampleTime "Timer Sample Time:"
      mask init:
      | block = gcb;
      | maskObj = Simulink.Mask.get(block);
      | maskObj.Display = sprintf('disp([''%s'' newline newline ''%s'']);', PLCBlockType, PLCOperandTag);
      | slplc.callbacks.initInstruction(block);
      settings: AttributesFormatString=%<PLCBlockType>: %<PLCOperandTag>
      mask Help: web([docroot '/plccoder/ref/ton' '.html']);
      mask DialogControl PLCBlockTitle Prompt: Timer On Delay (TON)
      mask Display: disp(['TON' newline newline 'TBIgnore']);
  TON1 : Subsystem  Priority=12  TreatAsAtomicUnit=on  mask{PLCOperandTag=T2, PLCTimerSampleTime=2000, PLCBlockType=TON, PLCPOUType=stdFB, PLCOperandAccess=ReadWrite, PLCOperandExpression=xxx_PLC_VAR_T2}
      mask prompts: PLCOperandTag "Timer Tag:"; PLCTimerSampleTime "Timer Sample Time:"
      mask init:
      | block = gcb;
      | maskObj = Simulink.Mask.get(block);
      | maskObj.Display = sprintf('disp([''%s'' newline newline ''%s'']);', PLCBlockType, PLCOperandTag);
      | slplc.callbacks.initInstruction(block);
      settings: AttributesFormatString=%<PLCBlockType>: %<PLCOperandTag>
      mask Help: web([docroot '/plccoder/ref/ton' '.html']);
      mask DialogControl PLCBlockTitle Prompt: Timer On Delay (TON)
      mask Display: disp(['TON' newline newline 'T2']);
  TON3 : Subsystem  Priority=16  TreatAsAtomicUnit=on  mask{PLCOperandTag=T3, PLCTimerSampleTime=2000, PLCBlockType=TON, PLCPOUType=stdFB, PLCOperandAccess=ReadWrite, PLCOperandExpression=xxx_PLC_VAR_T3}
      mask prompts: PLCOperandTag "Timer Tag:"; PLCTimerSampleTime "Timer Sample Time:"
      mask init:
      | block = gcb;
      | maskObj = Simulink.Mask.get(block);
      | maskObj.Display = sprintf('disp([''%s'' newline newline ''%s'']);', PLCBlockType, PLCOperandTag);
      | slplc.callbacks.initInstruction(block);
      settings: AttributesFormatString=%<PLCBlockType>: %<PLCOperandTag>
      mask Help: web([docroot '/plccoder/ref/ton' '.html']);
      mask DialogControl PLCBlockTitle Prompt: Timer On Delay (TON)
      mask Display: disp(['TON' newline newline 'T3']);
  TON4 : Subsystem  Priority=8  TreatAsAtomicUnit=on  mask{PLCOperandTag=T1, PLCTimerSampleTime=2000, PLCBlockType=TON, PLCPOUType=stdFB, PLCOperandAccess=ReadWrite, PLCOperandExpression=xxx_PLC_VAR_T1}
      mask prompts: PLCOperandTag "Timer Tag:"; PLCTimerSampleTime "Timer Sample Time:"
      mask init:
      | block = gcb;
      | maskObj = Simulink.Mask.get(block);
      | maskObj.Display = sprintf('disp([''%s'' newline newline ''%s'']);', PLCBlockType, PLCOperandTag);
      | slplc.callbacks.initInstruction(block);
      settings: AttributesFormatString=%<PLCBlockType>: %<PLCOperandTag>
      mask Help: web([docroot '/plccoder/ref/ton' '.html']);
      mask DialogControl PLCBlockTitle Prompt: Timer On Delay (TON)
      mask Display: disp(['TON' newline newline 'T1']);
  Up to Parent POU : Subsystem  DisableCoverage=on  TreatAsAtomicUnit=on  mask{PLCBlockType=OpenParentPOU}
      settings: OpenFcn=slplc.callbacks.openParentPOUBlock(gcb);
      mask Help: web([docroot '/plccoder/ref/uptoparentpou' '.html']);
      mask DialogControl PLCBlockTitle Prompt: Add Single Rung
  XIC : Subsystem  Priority=18  TreatAsAtomicUnit=on  mask{PLCOperandTag=BIgnore, PLCBlockType=XIC, PLCPOUType=Contact, PLCOperandExpression=xxx_PLC_VAR_BIgnore}
      mask prompts: PLCOperandTag "Operand Tag:"
      mask init:
      | slplc.callbacks.initInstruction(gcb);
      settings: AttributesFormatString=%<PLCOperandTag>
      mask Help: web([docroot '/plccoder/ref/xic' '.html']);
      mask DialogControl PLCBlockTitle Prompt: Examine If Closed (XIC)
  XIC1 : Subsystem  Priority=10  TreatAsAtomicUnit=on  mask{PLCOperandTag=B, PLCBlockType=XIC, PLCPOUType=Contact, PLCOperandExpression=xxx_PLC_VAR_B}
      mask prompts: PLCOperandTag "Operand Tag:"
      mask init:
      | slplc.callbacks.initInstruction(gcb);
      settings: AttributesFormatString=%<PLCOperandTag>
      mask Help: web([docroot '/plccoder/ref/xic' '.html']);
      mask DialogControl PLCBlockTitle Prompt: Examine If Closed (XIC)
  XIC10 : Subsystem  Priority=48  TreatAsAtomicUnit=on  mask{PLCOperandTag=TBIgnore.DN, PLCBlockType=XIC, PLCPOUType=Contact, PLCOperandExpression=xxx_PLC_VAR_TBIgnore.DN}
      mask prompts: PLCOperandTag "Operand Tag:"
      mask init:
      | slplc.callbacks.initInstruction(gcb);
      settings: AttributesFormatString=%<PLCOperandTag>
      mask Help: web([docroot '/plccoder/ref/xic' '.html']);
      mask DialogControl PLCBlockTitle Prompt: Examine If Closed (XIC)
  XIC11 : Subsystem  Priority=6  TreatAsAtomicUnit=on  mask{PLCOperandTag=A, PLCBlockType=XIC, PLCPOUType=Contact, PLCOperandExpression=xxx_PLC_VAR_A}
      mask prompts: PLCOperandTag "Operand Tag:"
      mask init:
      | slplc.callbacks.initInstruction(gcb);
      settings: AttributesFormatString=%<PLCOperandTag>
      mask Help: web([docroot '/plccoder/ref/xic' '.html']);
      mask DialogControl PLCBlockTitle Prompt: Examine If Closed (XIC)
  XIC2 : Subsystem  Priority=21  TreatAsAtomicUnit=on  mask{PLCOperandTag=T1.DN, PLCBlockType=XIC, PLCPOUType=Contact, PLCOperandExpression=xxx_PLC_VAR_T1.DN}
      mask prompts: PLCOperandTag "Operand Tag:"
      mask init:
      | slplc.callbacks.initInstruction(gcb);
      settings: AttributesFormatString=%<PLCOperandTag>
      mask Help: web([docroot '/plccoder/ref/xic' '.html']);
      mask DialogControl PLCBlockTitle Prompt: Examine If Closed (XIC)
  XIC3 : Subsystem  Priority=31  TreatAsAtomicUnit=on  mask{PLCOperandTag=T2.DN, PLCBlockType=XIC, PLCPOUType=Contact, PLCOperandExpression=xxx_PLC_VAR_T2.DN}
      mask prompts: PLCOperandTag "Operand Tag:"
      mask init:
      | slplc.callbacks.initInstruction(gcb);
      settings: AttributesFormatString=%<PLCOperandTag>
      mask Help: web([docroot '/plccoder/ref/xic' '.html']);
      mask DialogControl PLCBlockTitle Prompt: Examine If Closed (XIC)
  XIC4 : Subsystem  Priority=3  TreatAsAtomicUnit=on  mask{PLCOperandTag=Button, PLCBlockType=XIC, PLCPOUType=Contact, PLCOperandExpression=xxx_PLC_VAR_Button}
      mask prompts: PLCOperandTag "Operand Tag:"
      mask init:
      | slplc.callbacks.initInstruction(gcb);
      settings: AttributesFormatString=%<PLCOperandTag>
      mask Help: web([docroot '/plccoder/ref/xic' '.html']);
      mask DialogControl PLCBlockTitle Prompt: Examine If Closed (XIC)
  XIC6 : Subsystem  Priority=25  TreatAsAtomicUnit=on  mask{PLCOperandTag=ButtonLatch, PLCBlockType=XIC, PLCPOUType=Contact, PLCOperandExpression=xxx_PLC_VAR_ButtonLatch}
      mask prompts: PLCOperandTag "Operand Tag:"
      mask init:
      | slplc.callbacks.initInstruction(gcb);
      settings: AttributesFormatString=%<PLCOperandTag>
      mask Help: web([docroot '/plccoder/ref/xic' '.html']);
      mask DialogControl PLCBlockTitle Prompt: Examine If Closed (XIC)
  XIC7 : Subsystem  Priority=35  TreatAsAtomicUnit=on  mask{PLCOperandTag=ButtonLatch, PLCBlockType=XIC, PLCPOUType=Contact, PLCOperandExpression=xxx_PLC_VAR_ButtonLatch}
      mask prompts: PLCOperandTag "Operand Tag:"
      mask init:
      | slplc.callbacks.initInstruction(gcb);
      settings: AttributesFormatString=%<PLCOperandTag>
      mask Help: web([docroot '/plccoder/ref/xic' '.html']);
      mask DialogControl PLCBlockTitle Prompt: Examine If Closed (XIC)
  XIC8 : Subsystem  Priority=14  TreatAsAtomicUnit=on  mask{PLCOperandTag=C, PLCBlockType=XIC, PLCPOUType=Contact, PLCOperandExpression=xxx_PLC_VAR_C}
      mask prompts: PLCOperandTag "Operand Tag:"
      mask init:
      | slplc.callbacks.initInstruction(gcb);
      settings: AttributesFormatString=%<PLCOperandTag>
      mask Help: web([docroot '/plccoder/ref/xic' '.html']);
      mask DialogControl PLCBlockTitle Prompt: Examine If Closed (XIC)
  XIC9 : Subsystem  Priority=42  TreatAsAtomicUnit=on  mask{PLCOperandTag=T3.DN, PLCBlockType=XIC, PLCPOUType=Contact, PLCOperandExpression=xxx_PLC_VAR_T3.DN}
      mask prompts: PLCOperandTag "Operand Tag:"
      mask init:
      | slplc.callbacks.initInstruction(gcb);
      settings: AttributesFormatString=%<PLCOperandTag>
      mask Help: web([docroot '/plccoder/ref/xic' '.html']);
      mask DialogControl PLCBlockTitle Prompt: Examine If Closed (XIC)
  XIO : Subsystem  Priority=22  TreatAsAtomicUnit=on  mask{PLCOperandExpression=xxx_PLC_VAR_ButtonLatch, PLCOperandTag=ButtonLatch, PLCBlockType=XIO, PLCPOUType=Contact}
      mask prompts: PLCOperandTag "Operand Tag:"
      mask init:
      | slplc.callbacks.initInstruction(gcb);
      settings: AttributesFormatString=%<PLCOperandTag>
      mask Help: web([docroot '/plccoder/ref/xio' '.html']);
      mask DialogControl PLCBlockTitle Prompt: Examine If Open (XIO)
  XIO1 : Subsystem  Priority=2  TreatAsAtomicUnit=on  mask{PLCOperandExpression=xxx_PLC_VAR_BIgnore, PLCOperandTag=BIgnore, PLCBlockType=XIO, PLCPOUType=Contact}
      mask prompts: PLCOperandTag "Operand Tag:"
      mask init:
      | slplc.callbacks.initInstruction(gcb);
      settings: AttributesFormatString=%<PLCOperandTag>
      mask Help: web([docroot '/plccoder/ref/xio' '.html']);
      mask DialogControl PLCBlockTitle Prompt: Examine If Open (XIO)
  XIO2 : Subsystem  Priority=32  TreatAsAtomicUnit=on  mask{PLCOperandExpression=xxx_PLC_VAR_ButtonLatch, PLCOperandTag=ButtonLatch, PLCBlockType=XIO, PLCPOUType=Contact}
      mask prompts: PLCOperandTag "Operand Tag:"
      mask init:
      | slplc.callbacks.initInstruction(gcb);
      settings: AttributesFormatString=%<PLCOperandTag>
      mask Help: web([docroot '/plccoder/ref/xio' '.html']);
      mask DialogControl PLCBlockTitle Prompt: Examine If Open (XIO)
  wires:
  XIC1/1(RungOut) -> OTE1/1(RungIn)
  TON1/1(EN) -> Rung Terminal6/1(RungIn)
  OTL/1(RungOut) -> OTU/1(RungIn)
  XIC2/1(RungOut) -> XIC6/1(RungIn), XIO/1(RungIn)
  Junction/1(RungOut) -> Rung Terminal3/1(RungIn)
  OTE1/1(RungOut) -> TON1/1(RungIn)
  XIC4/1(RungOut) -> OTL1/1(RungIn)
  XIO/1(RungOut) -> OTL/1(RungIn)
  XIC6/1(RungOut) -> OTU2/1(RungIn)
  OTU2/1(RungOut) -> OTU3/1(RungIn)
  OTU3/1(RungOut) -> OTL2/1(RungIn)
  OTL2/1(RungOut) -> Junction/2(RungIn2)
  OTU/1(RungOut) -> Junction/1(RungIn1)
  OTU1/1(RungOut) -> Junction1/1(RungIn1)
  XIC7/1(RungOut) -> OTU4/1(RungIn)
  OTL3/1(RungOut) -> OTU1/1(RungIn)
  OTU4/1(RungOut) -> OTU5/1(RungIn)
  OTL4/1(RungOut) -> OTU6/1(RungIn)
  OTU5/1(RungOut) -> OTL4/1(RungIn)
  XIC3/1(RungOut) -> XIO2/1(RungIn), XIC7/1(RungIn)
  Junction1/1(RungOut) -> Rung Terminal4/1(RungIn)
  XIO2/1(RungOut) -> OTL3/1(RungIn)
  OTU6/1(RungOut) -> Junction1/2(RungIn2)
  XIC9/1(RungOut) -> OTL5/1(RungIn)
  OTL5/1(RungOut) -> OTL6/1(RungIn)
  Power Rail Start/1(PowerOut) -> XIO1/1(RungIn), XIC11/1(RungIn), XIC8/1(RungIn), XIC/1(RungIn), XIC9/1(RungIn), XIC10/1(RungIn), Power Rail Terminal/1(PowerIn), XIC3/1(RungIn), XIC2/1(RungIn), XIC1/1(RungIn)
  XIO1/1(RungOut) -> XIC4/1(RungIn)
  OTL6/1(RungOut) -> OTU7/1(RungIn)
  XIC10/1(RungOut) -> OTU8/1(RungIn)
  OTU8/1(RungOut) -> Rung Terminal9/1(RungIn)
  OTE4/1(RungOut) -> TON4/1(RungIn)
  XIC11/1(RungOut) -> OTE4/1(RungIn)
  OTU7/1(RungOut) -> OTU9/1(RungIn)
  OTU9/1(RungOut) -> Rung Terminal8/1(RungIn)
  TON3/1(EN) -> Rung Terminal7/1(RungIn)
  XIC8/1(RungOut) -> OTE3/1(RungIn)
  OTE3/1(RungOut) -> TON3/1(RungIn)
  XIC/1(RungOut) -> TON/1(RungIn)
  TON/1(EN) -> Rung Terminal2/1(RungIn)
  TON4/1(EN) -> Rung Terminal10/1(RungIn)
  OTL1/1(RungOut) -> Rung Terminal1/1(RungIn)
